simulink model "dspwprf"  (Simulink 5.0)
settings: Solver=FixedStepDiscrete  StartTime=0.0  StopTime=1024  RelTol=1e-3
PreLoadFcn:
  | load dspwlets;
values from neighbouring files (symbols this model uses):
  ts = [-1 0]    [lmsxy.m]    (also in sdspwwvdisp.m = get_param(blk,'CompiledSampleTime'))
undefined symbols (not defined in the file or in its folder): lod
libraries: dspsigops x3, dspsnks4 x3, dspmlti4 x2, dspsrcs4 x1
settings Model: Creator=don  LastModifiedBy=mkhan  ExtModeTrigMode=oneshot  ExtModeArmWhenConnect=off  SaveTime=off  SaveOutput=off  LimitDataPoints=off  IntegerOverflowMsg=none  RTWInlineParameters=on  BlockReductionOpt=off  BooleanDataType=off  ZeroCrossControl=UseLocalSettings  TargetHWChar=2  TargetHWWordLengths=8,16,32,32  RTWMathFcnLibMatFile=iso_c_tmw.mat  RTWOptions="-aEnforceIntegerDowncast=1 -aFoldNonRolledExpr=1 -aInlineInvariantSignals=1 -aInlineParameters=1 -aLocalBlockOutputs=1 -aRollThreshold=2 -aRTWVerbose=1 -aForceParamTrailComments=0 -aGenerateComments=1 -aIgnoreCustomStorageClasses=1 -aIncHierarchyInIds=0 -aMaxRTWIdLen=31 -aShowEliminatedStatements=0 -aReadOnly=0 -aTargetFcnLib=\"iso_c_tmw.mat\" -aIncDataTypeInIds=0 -aPrefixModelToSubsysFcnNames=1 -aInlinedPrmAccess=\"Literals\" -aGenerateFullHeader=1 -aIsPILTarget=0 -aGenerateReport=0 -aLogVarNameModifier=\"rt_\" -aExtMode=0 -aExtModeStaticAlloc=0 -aExtModeTesting=0 -aExtModeStaticAllocSize=1000000 -aExtModeTransport=0"

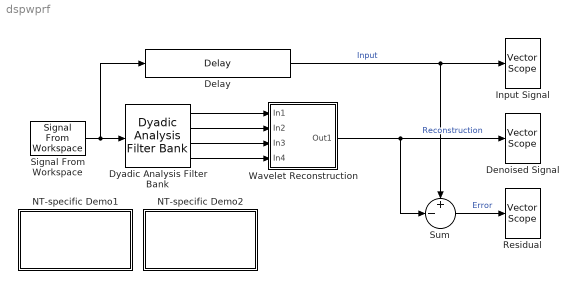
== system dspwprf ==
  Delay : dspsigops/Delay  dly_unit=Samples  delay=7*(length(lod)-1)  ic_detail=on  dif_ic_for_ch=off  dif_ic_for_dly=off  ic=0  reset_popup=None
  Denoised Signal : dspsnks4/Vector Scope  ScopeProperties=on  Domain=Time  HorizSpan=15  DisplayProperties=off  AxisGrid=on  Memory=off  FrameNumber=on  AxisLegend=off  AxisZoom=off  OpenScopeAtSimStart=on  OpenScopeImmediately=off  FigPos=[720 345 430 200]  AxisProperties=off  XUnits=Hertz  XRange=[0...Fs/2]  InheritXIncr=on  XIncr=1  XLabel=Samples  YUnits=dB  YLabel=Amplitude  LineProperties=off
      settings: YMin=-10  YMax=10
  Dyadic Analysis Filter Bank : dspmlti4/Dyadic Analysis Filter Bank  Wname=User-defined  OrdRec_ordDec=[1 / 1]  Order=2  LPF=lod  HPF=hid  NumLevels=3  tree=Asymmetric  Output=Multiple ports
  Input Signal : dspsnks4/Vector Scope  ScopeProperties=on  Domain=Time  HorizSpan=15  DisplayProperties=off  AxisGrid=on  Memory=off  FrameNumber=on  AxisLegend=off  AxisZoom=off  OpenScopeAtSimStart=on  OpenScopeImmediately=off  FigPos=[720 590 430 200]  AxisProperties=off  XUnits=Hertz  XRange=[0...Fs/2]  InheritXIncr=on  XIncr=1  XLabel=Samples  YUnits=dB  YLabel=Amplitude  LineProperties=off
      settings: YMin=-10  YMax=10
  NT-specific Demo1 : Subsystem
      settings: OpenFcn=dspwpr
      mask Type: Sample-Based Demo
      mask Display: disp('Sample-Based\nDemo')
  NT-specific Demo2 : Subsystem
      settings: OpenFcn=dspwprfp
      mask Type: Fixed-Point Demo
      mask Display: disp('Fixed-Point\nDemo')
  Residual : dspsnks4/Vector Scope  ScopeProperties=on  Domain=Time  HorizSpan=15  DisplayProperties=off  AxisGrid=on  Memory=off  FrameNumber=on  AxisLegend=off  AxisZoom=off  OpenScopeAtSimStart=on  OpenScopeImmediately=off  FigPos=[720 100 430 200]  AxisProperties=off  XUnits=Hertz  XRange=[0...Fs/2]  InheritXIncr=on  XIncr=1  XLabel=Samples  YUnits=dB  YLabel=Amplitude  LineProperties=off
      settings: YMin=-3.00160967239117  YMax=2.37514789840845
  Signal From Workspace : dspsrcs4/Signal From Workspace  X=noisdopp  Ts=ts  nsamps=64  OutputAfterFinalValue=Setting to zero
  Sum : Sum  Inputs=+-|  SaturateOnIntegerOverflow=on  InputSameDT=on
  Wavelet Reconstruction : Subsystem
  wires:
  Signal From Workspace/1 -> Dyadic Analysis Filter Bank/1, Delay/1
  Dyadic Analysis Filter Bank/4 -> Wavelet Reconstruction/4(In4)
  Dyadic Analysis Filter Bank/3 -> Wavelet Reconstruction/3(In3)
  Dyadic Analysis Filter Bank/2 -> Wavelet Reconstruction/2(In2)
  Dyadic Analysis Filter Bank/1 -> Wavelet Reconstruction/1(In1)
  Wavelet Reconstruction/1(Out1) -> Sum/2, Denoised Signal/1  "Reconstruction"
  Sum/1 -> Residual/1  "Error"
  Delay/1 -> Sum/1, Input Signal/1  "Input"

== system dspwprf/NT-specific Demo1 ==

== system dspwprf/NT-specific Demo2 ==

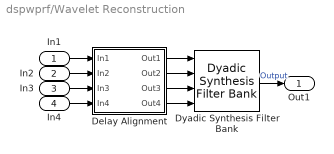
== system dspwprf/Wavelet Reconstruction ==
  In1 : Inport
  In2 : Inport  Port=2
  In3 : Inport  Port=3
  In4 : Inport  Port=4
  Delay Alignment : Subsystem
  Dyadic Synthesis Filter Bank : dspmlti4/Dyadic Synthesis Filter Bank  Wname=User-defined  OrdRec_ordDec=[1 / 1]  Order=2  LPF=lor  HPF=hir  NumLevels=3  tree=Asymmetric  Input=Multiple ports
  Out1 : Outport
  wires:
  Delay Alignment/1(Out1) -> Dyadic Synthesis Filter Bank/1
  Delay Alignment/2(Out2) -> Dyadic Synthesis Filter Bank/2
  Delay Alignment/3(Out3) -> Dyadic Synthesis Filter Bank/3
  Delay Alignment/4(Out4) -> Dyadic Synthesis Filter Bank/4
  In1/1 -> Delay Alignment/1(In1)
  In2/1 -> Delay Alignment/2(In2)
  Dyadic Synthesis Filter Bank/1 -> Out1/1  "Output"
  In3/1 -> Delay Alignment/3(In3)
  In4/1 -> Delay Alignment/4(In4)

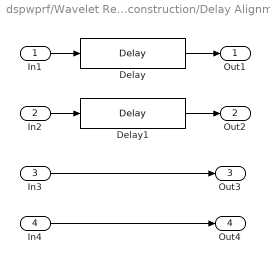
== system dspwprf/Wavelet Reconstruction/Delay Alignment ==
  In1 : Inport
  In2 : Inport  Port=2
  In3 : Inport  Port=3
  In4 : Inport  Port=4
  Delay : dspsigops/Delay  dly_unit=Samples  delay=3*(length(lod)-1)  ic_detail=on  dif_ic_for_ch=off  dif_ic_for_dly=off  ic=0  reset_popup=None
  Delay1 : dspsigops/Delay  dly_unit=Samples  delay=length(lod) - 1  ic_detail=on  dif_ic_for_ch=off  dif_ic_for_dly=off  ic=0  reset_popup=None
  Out1 : Outport
  Out2 : Outport  Port=2
  Out3 : Outport  Port=3
  Out4 : Outport  Port=4
  wires:
  In3/1 -> Out3/1
  In4/1 -> Out4/1
  In2/1 -> Delay1/1
  Delay1/1 -> Out2/1
  In1/1 -> Delay/1
  Delay/1 -> Out1/1
